simulink model "dbx_control_v0_05"  (R2015a)
settings: Solver=FixedStepDiscrete  SolverMode=SingleTasking  StartTime=0.0  StopTime=20  FixedStep=T_ctrl  RelTol=1e-3
undefined symbols (not defined in the file): A_l_max_x, A_M, A_z_max, CG, epsilon, Flaps_ang_deg, g, Hover_eta_23, Hover_throtle_1, Hover_throtle_23, I_BAC, L_M, m, psi_f_i, psi_K_b, psi_tau, Roll_pich_sens, Servo_calib, T_ctrl, Throtle_sens, v_i0, Yaw_sens
libraries: DBX_model x29, DBX_Control_lib x15, simulink x9, DBX_Control x3
(part 2 of 2)

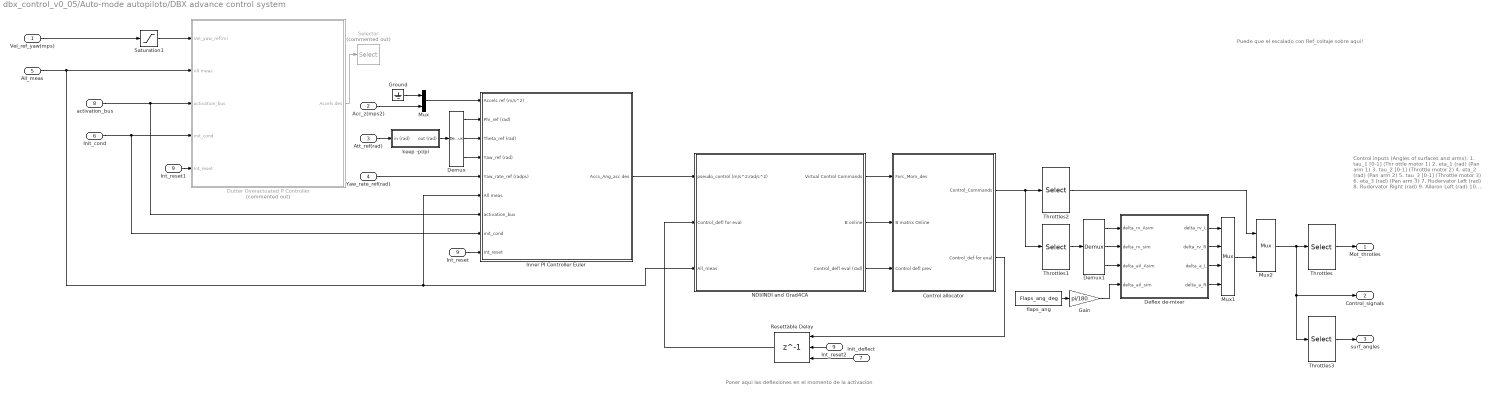
== system dbx_control_v0_05/Auto-mode autopiloto/DBX advance control system ==
  note: Puede que el escalado con Ref_coltaje sobre aqui!
  note: Poner aqui las deflexiones en el momento de la activacion
  note: Control inputs (Angles  of surfaces and arms):
      |
      | 1. tau_1 [0-1] (Thr ottle motor 1)
      | 2. eta_1 (rad)  (Pan arm 1)
      |
      | 3. tau_2 [0-1] (Throttle motor 2)
      | 4. eta_2 (rad)  (Pan arm 2)
      |
      | 5. tau_3 [0-1] (Throttle motor 3)
      | 6. eta_3 (rad)  (Pan arm  3)
      |
      | 7. Rudervator Left (rad)
      | 8. Rudervator Right (rad)
      | 9. Aileron Left (rad)
      | 10. Aielron Right (rad)
  Vel_ref_yaw(mps) : Inport
  Acc_z(mps2) : Inport  Port=2
  Att_ref(rad) : Inport  Port=3
  Yaw_rate_ref(rad) : Inport  Port=4
  All_meas : Inport  Port=5
  Init_cond : Inport  Port=6
  Init_deflect : Inport  Port=7  PortDimensions=[9,1]
  activation_bus : Inport  Port=8
  Int_reset : Inport  Port=9
  Control allocator : Subsystem  RTWFcnName=abc  RTWFileName=asas  VariantControl=Control Allocator: NO RECONFIG
      settings: MinAlgLoopOccurrences=on  RTWFcnNameOpts=User specified  RTWFileNameOpts=User specified
  Deflex de-mixer : Subsystem  TreatAsAtomicUnit=on
  Demux : Demux  Outputs=3
  Demux1 : Demux  Outputs=3
  Gain : Gain  Gain=pi/180
  Ground : Ground
  Inner PI Controller Euler : Subsystem  VariantControl=PI_quat
  Int_reset1 : InportShadow  Port=9
  Int_reset2 : InportShadow  Port=9
  Mux : Mux  Inputs=[2,1]
  Mux1 : Mux
  Mux2 : Mux  Inputs=[6,4]
  NDI/INDI and Grad4CA : Subsystem  Variant=on  VariantControl=NDI: NO RECONFIG  OverrideUsingVariant=NDI_incremental_grad
  Outter Overactuated P Controller : Subsystem  Commented=on  VariantControl=Overactuated P Controller
  Resettable Delay : Delay  DelayLength=1  InitialConditionSource=Input port  ExternalReset=Either  InputProcessing=Inherited  SampleTime=T_ctrl
      settings: InputPortMap=u0,r5,p4
  Saturation1 : Saturate  UpperLimit=[10,10,v_i0]'  LowerLimit=-[10,10,2*v_i0]'
  Selector : Selector  Commented=on  InputPortWidth=3  Indices=1:2
  Throttles : Selector  InputPortWidth=10  Indices=[1,3,5]
  Throttles1 : Selector  InputPortWidth=9  Indices=[7:9]
  Throttles2 : Selector  InputPortWidth=9  Indices=[1:6]
  Throttles3 : Selector  InputPortWidth=10  Indices=[2,4,6,7,8,9,10]
  flaps_ang : Constant  Value=Flaps_ang_deg  OutDataTypeStr=single
  keep -pi/pi : Subsystem
  Mot_throtles : Outport
  Control_signals : Outport  Port=2
  surf_angles : Outport  Port=3
  wires:
  All_meas/1 -> Inner PI Controller Euler/6(All meas), NDI/INDI and Grad4CA/3(All_meas), Outter Overactuated P Controller/2(All meas)
  NDI/INDI and Grad4CA/3(Control_defl eval (rad)) -> Control allocator/3(Control defl prev)
  keep -pi/pi/1(out (rad)) -> Demux/1
  Demux/3 -> Inner PI Controller Euler/4(Yaw_ref (rad))
  Demux/2 -> Inner PI Controller Euler/3(Theta_ref (rad))
  Demux/1 -> Inner PI Controller Euler/2(Phi_ref (rad))
  Att_ref(rad)/1 -> keep -pi/pi/1(in (rad))
  Throttles/1 -> Mot_throtles/1
  Control allocator/1(Control_Commands) -> Throttles1/1, Throttles2/1
  Resettable Delay/1 -> NDI/INDI and Grad4CA/2(Control_defl for eval)
  Vel_ref_yaw(mps)/1 -> Saturation1/1
  Saturation1/1 -> Outter Overactuated P Controller/1(Vel_yaw_ref(m))
  Init_cond/1 -> Inner PI Controller Euler/8(init_cond), Outter Overactuated P Controller/4(init_cond)
  activation_bus/1 -> Inner PI Controller Euler/7(activation_bus), Outter Overactuated P Controller/3(activation_bus)
  Control allocator/2(Control_def for eval) -> Resettable Delay/1
  NDI/INDI and Grad4CA/2(B online) -> Control allocator/2(B matrix Online)
  Inner PI Controller Euler/1(Accs_Ang_acc des) -> NDI/INDI and Grad4CA/1(pseudo_control (m/s^2;rad/s^2))
  Demux1/2 -> Deflex de-mixer/2(delta_rv_sim)
  Demux1/3 -> Deflex de-mixer/3(delta_ail_Asim)
  Demux1/1 -> Deflex de-mixer/1(delta_rv_Asim)
  Throttles1/1 -> Demux1/1
  Throttles2/1 -> Mux2/1
  Deflex de-mixer/1(delta_rv_L) -> Mux1/1
  Deflex de-mixer/2(delta_rv_R) -> Mux1/2
  Deflex de-mixer/3(delta_a_L) -> Mux1/3
  Deflex de-mixer/4(delta_a_R) -> Mux1/4
  Mux1/1 -> Mux2/2
  Mux2/1 -> Throttles3/1, Control_signals/1, Throttles/1
  Throttles3/1 -> surf_angles/1
  Yaw_rate_ref(rad)/1 -> Inner PI Controller Euler/5(Yaw_rate_ref (radps))
  Int_reset/1 -> Inner PI Controller Euler/9(Int_reset)
  Int_reset1/1 -> Outter Overactuated P Controller/5(Int_reset)
  Acc_z(mps2)/1 -> Mux/2
  Mux/1 -> Inner PI Controller Euler/1(Accels ref (m/s^2))
  Init_deflect/1 -> Resettable Delay/3
  Int_reset2/1 -> Resettable Delay/2
  NDI/INDI and Grad4CA/1(Virtual Control Commands) -> Control allocator/1(Forc_Mom_des)
  Outter Overactuated P Controller/1(Accels des) -> Selector/1
  Ground/1 -> Mux/1
  flaps_ang/1 -> Gain/1
  Gain/1 -> Deflex de-mixer/4(delta_ail_sim)

== system dbx_control_v0_05/Auto-mode autopiloto/Initial conditions ==
  All_meas : Inport
  Bus Creator1 : BusCreator  Inputs=6
  Bus Selector : BusSelector  OutputSignals=Meas.Eulr_meas_rad,Meas.omega_b_meas_radps
  Ground{,1..3} (4 alike) : Ground
  Init_cond : Outport
  wires:
  Ground2/1 -> Bus Creator1/3  "vel_yaw_xy_init"
  Bus Selector/2 -> Bus Creator1/6  "<omega_b_meas_radps>"
  Ground3/1 -> Bus Creator1/4  "vel_yaw_z_init"
  Bus Selector/1 -> Bus Creator1/5  "<Eulr_meas_rad>"
  Ground/1 -> Bus Creator1/1  "pos_xy_init"
  Ground1/1 -> Bus Creator1/2  "alt_init"
  All_meas/1 -> Bus Selector/1
  Bus Creator1/1 -> Init_cond/1

== system dbx_control_v0_05/Auto-mode autopiloto/Sensibilidades Radio ==
  Radio_in : Inport
  Demux : Demux
  Demux1 : Demux  Outputs=2
  Divide : Product  Inputs=**
  Divide1 : Product  Inputs=**
  Mux : Mux  Inputs=2
  Product : Product
  Saturation : Saturate  UpperLimit=9  LowerLimit=-5
  Throtle_sens : Constant  Value=Throtle_sens  OutDataTypeStr=single
  Unary Minus : UnaryMinus
  Yaw_sens : Constant  Value=Yaw_sens  OutDataTypeStr=single
  deg2rad : Gain  Gain=pi/180
  deg2rad1 : Gain  Gain=pi/180
  deg2rad2 : Gain  Gain=[1,-1]
  roll_pich_sens : Constant  Value=Roll_pich_sens  OutDataTypeStr=single
  Acc_z_mps2 : Outport
  Roll(rad) : Outport  Port=2
  Pitch(rad) : Outport  Port=3
  Yaw(radps) : Outport  Port=4
  wires:
  Demux/1 -> Product/1  "Throtle"
  Demux/2 -> Divide/1  "Yaw"
  Demux/3 -> Mux/2  "Pitch"
  Demux/4 -> Mux/1  "Roll"
  Radio_in/1 -> Demux/1
  Divide/1 -> Yaw(radps)/1
  Mux/1 -> Divide1/1
  Divide1/1 -> Demux1/1
  Demux1/1 -> Roll(rad)/1
  Demux1/2 -> Pitch(rad)/1
  Product/1 -> Saturation/1
  Saturation/1 -> Acc_z_mps2/1
  Yaw_sens/1 -> deg2rad/1
  deg2rad/1 -> Divide/2
  roll_pich_sens/1 -> deg2rad1/1
  deg2rad1/1 -> deg2rad2/1
  deg2rad2/1 -> Divide1/2
  Throtle_sens/1 -> Unary Minus/1
  Unary Minus/1 -> Product/2

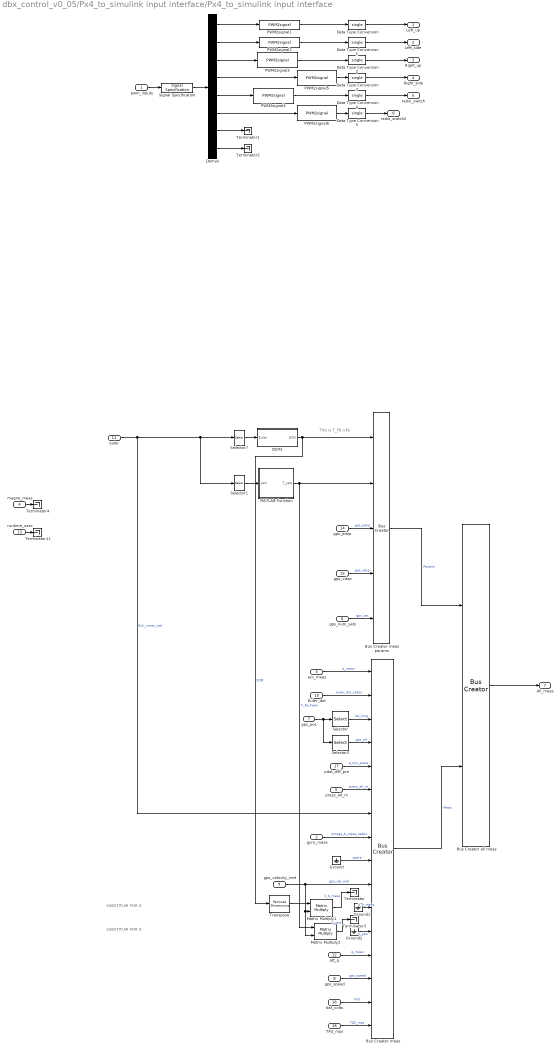
== system dbx_control_v0_05/Px4_to_simulink input interface/Px4_to_simulink input interface ==
  note: SUBSTITUIR POR 0
  note: This is T_Fb->Fe
  note: SUBSTITUIR POR 0
  pwm_inputs : Inport  PortDimensions=8  SampleTime=T_ctrl
  gyro_meas : Inport  Port=2  PortDimensions=3  SampleTime=T_ctrl
  acc_meas : Inport  Port=3  PortDimensions=3  SampleTime=T_ctrl
  magne_meas : Inport  Port=4  PortDimensions=3  SampleTime=T_ctrl
  press_alt_m : Inport  Port=5  PortDimensions=1  SampleTime=T_ctrl
  gps_num_sats : Inport  Port=6  PortDimensions=1  SampleTime=T_ctrl
  gps_pos : Inport  Port=7  PortDimensions=3  SampleTime=T_ctrl
  gps_speed : Inport  Port=8  PortDimensions=1  SampleTime=T_ctrl
  gps_velocity_ned : Inport  Port=9  PortDimensions=3  SampleTime=T_ctrl
  Euler_dot : Inport  Port=10  PortDimensions=3  SampleTime=T_ctrl
  euler : Inport  Port=11  PortDimensions=3  SampleTime=T_ctrl
  att_q : Inport  Port=12  PortDimensions=4  SampleTime=T_ctrl
  runtime_usec : Inport  Port=13  PortDimensions=1  SampleTime=T_ctrl
  gps_pdop : Inport  Port=14  PortDimensions=1  SampleTime=T_ctrl
  gps_vdop : Inport  Port=15  PortDimensions=1  SampleTime=T_ctrl
  bat_volts : Inport  Port=16  PortDimensions=1  SampleTime=T_ctrl
  pitot_diff_pre : Inport  Port=17  SampleTime=T_ctrl
  TAS_mps : Inport  Port=18  SampleTime=T_ctrl
  Bus Creator all meas : BusCreator  Inputs=2
  Bus Creator meas : BusCreator  Inputs=16
  Bus Creator meas params : BusCreator  Inputs=5
  DCM1 : Subsystem  TreatAsAtomicUnit=on
  Data Type Conversion{,1..5} (6 alike) : DataTypeConversion  OutDataTypeStr=single
  Demux : Demux  Outputs=8
  Ground : Ground
  Ground1 : Ground
  Ground2 : Ground
  MATLAB Function : MATLAB Function  TreatAsAtomicUnit=on
  Matrix Multiply1 : Product  Multiplication=Matrix(*)
  Matrix Multiply2 : Product  Multiplication=Matrix(*)
  PWM2signal{1..6} (6 alike) : DBX_model/PWM2signal  c=2000  a=1000  d=1  b=-1
  Selector : Selector  InputPortWidth=3  Indices=[1,2]
  Selector1 : Selector  InputPortWidth=3  Indices=3
  Selector2 : Selector  InputPortWidth=3  Indices=3
  Selector7 : Selector  InputPortWidth=3  Indices=[3 2 1]
  Signal Specification : SignalSpecification  Dimensions=8
  Terminator{,1..4,11} (6 alike) : Terminator
  Transpose : PermuteDimensions
  Left_up : Outport
  Left_side : Outport  Port=2
  Right_up : Outport  Port=3
  Right_side : Outport  Port=4
  radio_switch : Outport  Port=5
  radio_siwtch2 : Outport  Port=6
  All_meas : Outport  Port=7
  wires:
  PWM2signal1/1 -> Data Type Conversion/1
  PWM2signal2/1 -> Data Type Conversion1/1
  PWM2signal3/1 -> Data Type Conversion2/1
  PWM2signal5/1 -> Data Type Conversion3/1
  Bus Creator all meas/1 -> All_meas/1
  PWM2signal4/1 -> Data Type Conversion4/1
  att_q/1 -> Bus Creator meas/13  "q_meas"
  euler/1 -> Bus Creator meas/7, Selector1/1, Selector7/1  "Eulr_meas_rad"
  Euler_dot/1 -> Bus Creator meas/2  "euler_dot_radps"
  bat_volts/1 -> Bus Creator meas/15  "Volt"
  Bus Creator meas/1 -> Bus Creator all meas/2  "Meas"
  Bus Creator meas params/1 -> Bus Creator all meas/1  "Params"
  DCM1/1(DCM) -> Transpose/1, Bus Creator meas params/1  "DCM"
  acc_meas/1 -> Bus Creator meas/1  "a_meas"
  gps_pdop/1 -> Bus Creator meas params/3  "gps_pdop"
  gps_num_sats/1 -> Bus Creator meas params/5  "gps_sat"
  gps_vdop/1 -> Bus Creator meas params/4  "gps_vdop"
  Selector7/1 -> DCM1/1(Euler)
  Selector1/1 -> MATLAB Function/1(yaw)
  MATLAB Function/1(T_yaw) -> Matrix Multiply2/1, Bus Creator meas params/2  "T_Fe_Fyaw"
  Demux/1 -> PWM2signal1/1
  Demux/2 -> PWM2signal2/1
  Demux/3 -> PWM2signal3/1
  Demux/4 -> PWM2signal5/1
  Demux/5 -> PWM2signal4/1
  pwm_inputs/1 -> Signal Specification/1
  Demux/6 -> PWM2signal6/1
  Demux/7 -> Terminator1/1
  Demux/8 -> Terminator2/1
  gyro_meas/1 -> Bus Creator meas/8  "omega_b_meas_radps"
  magne_meas/1 -> Terminator4/1
  press_alt_m/1 -> Bus Creator meas/6  "press_alt_m"
  gps_pos/1 -> Selector2/1, Selector/1
  gps_speed/1 -> Bus Creator meas/14  "gps_speed"
  gps_velocity_ned/1 -> Bus Creator meas/10, Matrix Multiply1/2, Matrix Multiply2/2  "gps_vel_ned"
  runtime_usec/1 -> Terminator11/1
  Signal Specification/1 -> Demux/1
  PWM2signal6/1 -> Data Type Conversion5/1
  pitot_diff_pre/1 -> Bus Creator meas/5  "q_dyn_press"
  Selector/1 -> Bus Creator meas/3  "lat_long"
  Selector2/1 -> Bus Creator meas/4  "gps_alt"
  TAS_mps/1 -> Bus Creator meas/16  "TAS_mps"
  Transpose/1 -> Matrix Multiply1/1
  Ground1/1 -> Bus Creator meas/11  "V_b_meas"
  Ground2/1 -> Bus Creator meas/12  "V_yaw"
  Ground/1 -> Bus Creator meas/9  "spare"
  Matrix Multiply1/1 -> Terminator/1  "V_b_meas"
  Matrix Multiply2/1 -> Terminator3/1  "V_yaw"
  Data Type Conversion/1 -> Left_up/1
  Data Type Conversion1/1 -> Left_side/1
  Data Type Conversion2/1 -> Right_up/1
  Data Type Conversion3/1 -> Right_side/1
  Data Type Conversion4/1 -> radio_switch/1
  Data Type Conversion5/1 -> radio_siwtch2/1

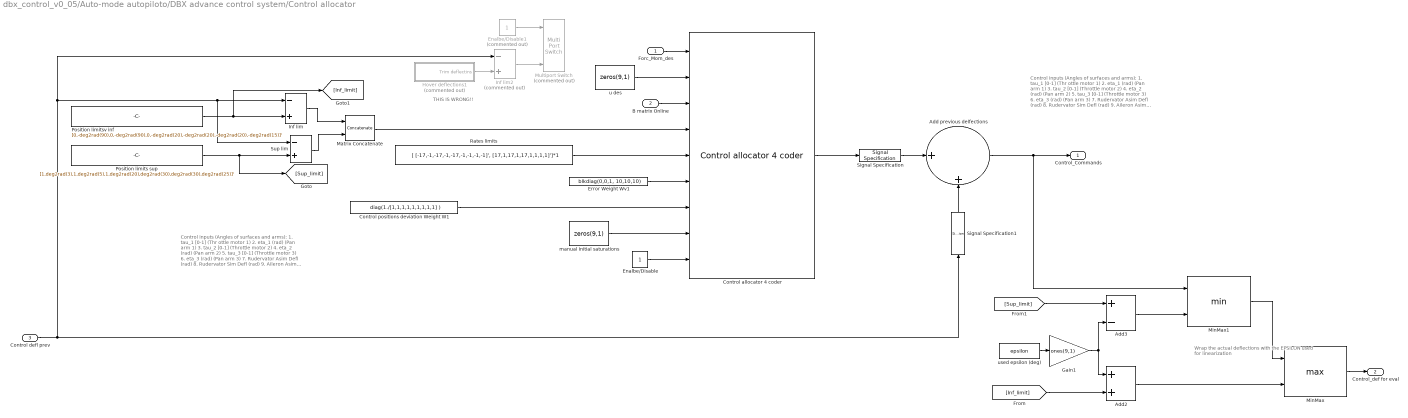
== system dbx_control_v0_05/Auto-mode autopiloto/DBX advance control system/Control allocator ==
  note: THIS IS WRONG!!
  note: Wrap the actual deflections with the EPSILON
      |  used for linearization
  note: Control inputs (Angles  of surfaces and arms):
      |
      | 1. tau_1 [0-1] (Thr ottle motor 1)
      | 2. eta_1 (rad)  (Pan arm 1)
      |
      | 3. tau_2 [0-1] (Throttle motor 2)
      | 4. eta_2 (rad)  (Pan arm 2)
      |
      | 5. tau_3 [0-1] (Throttle motor 3)
      | 6. eta_3 (rad)  (Pan arm  3)
      |
      | 7. Rudervator Asim Defl (rad)
      | 8. Rudervator Sim Defl (rad)
      | 9. Aileron Asim Defl (rad)
  note: Control inputs (Angles  of surfaces and arms):
      |
      | 1. tau_1 [0-1] (Thr ottle motor 1)
      | 2. eta_1 (rad)  (Pan arm 1)
      |
      | 3. tau_2 [0-1] (Throttle motor 2)
      | 4. eta_2 (rad)  (Pan arm 2)
      |
      | 5. tau_3 [0-1] (Throttle motor 3)
      | 6. eta_3 (rad)  (Pan arm  3)
      |
      | 7. Rudervator Asim Defl (rad)
      | 8. Rudervator Sim Defl (rad)
      | 9. Aileron Asim Defl (rad)
  Forc_Mom_des : Inport
  B matrix Online : Inport  Port=2
  Control defl prev : Inport  Port=3
  Add previous delfections : Sum  Inputs=|++
  Add2 : Sum
  Add3 : Sum  Inputs=+-
  Control allocator 4 coder : DBX_Control_lib/Control allocator 4 coder  gamma=1  imax=20  T=T_ctrl
  Control positions deviation Weight W1 : Constant  Value=diag(1./[1,1,1,1,1,1,1,1,1] )  OutDataTypeStr=single
  Enalbe/Disable : Constant  OutDataTypeStr=single
  Enalbe/Disable1 : Constant  Commented=on
  Error Weight Wv1 : Constant  Value=blkdiag(0,0,1, 10,10,10)  OutDataTypeStr=single
  Gain1 : Gain  Gain=ones(9,1)
  Hover deflections1 : Subsystem  Commented=on  TreatAsAtomicUnit=on
  Inf lim : Sum  Inputs=-+
  Inf lim2 : Sum  Commented=on  Inputs=-+
  Matrix Concatenate : Concatenate  Mode=Multidimensional array  ConcatenateDimension=2
  MinMax : MinMax  Function=max  Inputs=2
  MinMax1 : MinMax  Inputs=2
  Multiport Switch : MultiPortSwitch  Commented=on  Inputs=2
  Position limits sup : Constant  Value=[1,deg2rad(3),1,deg2rad(5),1,deg2rad(20),deg2rad(30),deg2rad(30),deg2rad(25)]'  OutDataTypeStr=single
  Position limitsv inf : Constant  Value=[0,-deg2rad(90),0,-deg2rad(90),0,-deg2rad(20),-deg2rad(20),-deg2rad(20),-deg2rad(15)]'  OutDataTypeStr=single
  Rates limits : Constant  Value=[ [-17,-1,-17,-1,-17,-1,-1,-1,-1]', [17,1,17,1,17,1,1,1,1]']*1  OutDataTypeStr=single
  Signal Specification : SignalSpecification  OutDataTypeStr=single  Dimensions=[9,1]
  Signal Specification1 : SignalSpecification  OutDataTypeStr=single  Dimensions=[9,1]
  Sup lim : Sum  Inputs=-+
  manual Initial saturations : Constant  Value=zeros(9,1)  OutDataTypeStr=single
  u des : Constant  Value=zeros(9,1)  OutDataTypeStr=single
  used epsilon (deg) : Constant  Value=epsilon  OutDataTypeStr=single
  Control_Commands : Outport
  Control_def for eval : Outport  Port=2
  wires:
  MinMax1/1 -> MinMax/1
  Add3/1 -> MinMax1/2
  used epsilon (deg)/1 -> Gain1/1
  Gain1/1 -> Add3/2, Add2/1
  Add2/1 -> MinMax/2
  Control positions deviation Weight W1/1 -> Control allocator 4 coder/7
  Control allocator 4 coder/1 -> Signal Specification/1
  Enalbe/Disable/1 -> Control allocator 4 coder/9
  manual Initial saturations/1 -> Control allocator 4 coder/8
  Sup lim/1 -> Matrix Concatenate/2
  Inf lim/1 -> Matrix Concatenate/1
  Position limitsv inf/1 -> [Inf_limit], Inf lim/2
  Position limits sup/1 -> [Sup_limit], Sup lim/2
  Rates limits/1 -> Control allocator 4 coder/5
  Add previous delfections/1 -> Control_Commands/1, MinMax1/1
  B matrix Online/1 -> Control allocator 4 coder/3
  Signal Specification/1 -> Add previous delfections/1
  Signal Specification1/1 -> Add previous delfections/2
  Forc_Mom_des/1 -> Control allocator 4 coder/1
  Matrix Concatenate/1 -> Control allocator 4 coder/4
  Control defl prev/1 -> Inf lim2/1, Inf lim/1, Sup lim/1, Signal Specification1/1
  Inf lim2/1 -> Multiport Switch/3
  Hover deflections1/1(Trim deflectins) -> Inf lim2/2
  MinMax/1 -> Control_def for eval/1
  Error Weight Wv1/1 -> Control allocator 4 coder/6
  [Inf_limit] -> Add2/2
  [Sup_limit] -> Add3/1
  Enalbe/Disable1/1 -> Multiport Switch/1
  u des/1 -> Control allocator 4 coder/2

== system dbx_control_v0_05/Auto-mode autopiloto/DBX advance control system/Deflex de-mixer ==
  note: Control outputs:
      |
      | 7. Rudervator Left (rad)
      | 8. Rudervator Right (rad)
      | 9. Aileron Left (rad)
      | 10. Aielron Right (rad)
  delta_rv_Asim : Inport
  delta_rv_sim : Inport  Port=2
  delta_ail_Asim : Inport  Port=3
  delta_ail_sim : Inport  Port=4
  Add : Sum  Inputs=|++
  Add1 : Sum  Inputs=|-+
  Add2 : Sum  Inputs=|++
  Add3 : Sum  Inputs=|-+
  delta_rv_L : Outport
  delta_rv_R : Outport  Port=2
  delta_a_L : Outport  Port=3
  delta_a_R : Outport  Port=4
  wires:
  delta_rv_Asim/1 -> Add1/1, Add/1
  Add/1 -> delta_rv_L/1
  delta_rv_sim/1 -> Add1/2, Add/2
  Add1/1 -> delta_rv_R/1
  delta_ail_Asim/1 -> Add3/1, Add2/1
  Add2/1 -> delta_a_L/1
  delta_ail_sim/1 -> Add2/2, Add3/2
  Add3/1 -> delta_a_R/1

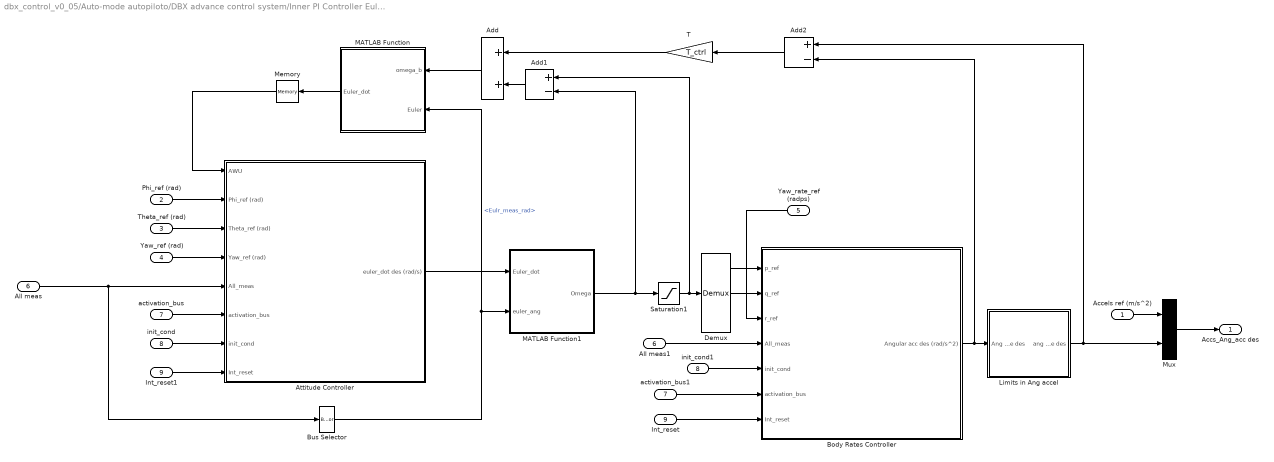
== system dbx_control_v0_05/Auto-mode autopiloto/DBX advance control system/Inner PI Controller Euler ==
  Accels ref (m/s^2) : Inport
  Phi_ref (rad) : Inport  Port=2
  Theta_ref (rad) : Inport  Port=3
  Yaw_ref (rad) : Inport  Port=4
  Yaw_rate_ref (radps) : Inport  Port=5
  All meas : Inport  Port=6
  activation_bus : Inport  Port=7
  init_cond : Inport  Port=8
  Int_reset : Inport  Port=9
  Add : Sum
  Add1 : Sum  Inputs=+-
  Add2 : Sum  Inputs=+-
  All meas1 : InportShadow  Port=6
  Attitude Controller : Subsystem
  Body Rates Controller : Subsystem
  Bus Selector : BusSelector  OutputSignals=Meas.Eulr_meas_rad
  Demux : Demux  Outputs=3
  Int_reset1 : InportShadow  Port=9
  Limits in Ang accel : Subsystem
  MATLAB Function : MATLAB Function
  MATLAB Function1 : MATLAB Function
  Memory : Memory
  Mux : Mux  Inputs=2
  Saturation1 : Saturate  UpperLimit=deg2rad(400)*[1,1,1]'  LowerLimit=-deg2rad(400)*[1,1,1]'
  T : Gain  Gain=T_ctrl
  activation_bus1 : InportShadow  Port=7
  init_cond1 : InportShadow  Port=8
  Accs_Ang_acc des : Outport
  wires:
  Accels ref (m/s^2)/1 -> Mux/1
  Mux/1 -> Accs_Ang_acc des/1
  All meas/1 -> Bus Selector/1, Attitude Controller/5(All_meas)
  Bus Selector/1 -> MATLAB Function/2(Euler), MATLAB Function1/2(euler_ang)  "<Eulr_meas_rad>"
  Demux/1 -> Body Rates Controller/1(p_ref)
  Demux/2 -> Body Rates Controller/2(q_ref)
  Phi_ref (rad)/1 -> Attitude Controller/2(Phi_ref (rad))
  Yaw_ref (rad)/1 -> Attitude Controller/4(Yaw_ref (rad))
  Limits in Ang accel/1(ang Ace des) -> Add2/1, Mux/2
  MATLAB Function1/1(Omega) -> Add1/2, Saturation1/1
  Body Rates Controller/1(Angular acc des (rad/s^2)) -> Add2/2, Limits in Ang accel/1(Ang Ace des)
  Add/1 -> MATLAB Function/1(omega_b)
  Add2/1 -> T/1
  Add1/1 -> Add/2
  T/1 -> Add/1
  MATLAB Function/1(Euler_dot) -> Memory/1
  init_cond/1 -> Attitude Controller/7(init_cond)
  activation_bus/1 -> Attitude Controller/6(activation_bus)
  All meas1/1 -> Body Rates Controller/4(All_meas)
  Saturation1/1 -> Add1/1, Demux/1
  Memory/1 -> Attitude Controller/1(AWU)
  Theta_ref (rad)/1 -> Attitude Controller/3(Theta_ref (rad))
  Attitude Controller/1(euler_dot des (rad/s)) -> MATLAB Function1/1(Euler_dot)
  Int_reset/1 -> Body Rates Controller/7(Int_reset)
  Int_reset1/1 -> Attitude Controller/8(Int_reset)
  activation_bus1/1 -> Body Rates Controller/6(activation_bus)
  init_cond1/1 -> Body Rates Controller/5(init_cond)
  Yaw_rate_ref (radps)/1 -> Body Rates Controller/3(r_ref)

== system dbx_control_v0_05/Auto-mode autopiloto/DBX advance control system/NDI//INDI and Grad4CA ==
  pseudo_control (m/s^2;rad/s^2) : Inport
  Control_defl for eval : Inport  Port=2
  All_meas : Inport  Port=3
  INDI and NDI : Subsystem  RTWFcnName=abc  RTWFileName=asas  VariantControl=NDI_INDI
      settings: RTWFcnNameOpts=User specified  RTWFileNameOpts=User specified
  NDI : Subsystem  RTWFcnName=abc  RTWFileName=asas  VariantControl=NDI
      settings: RTWFcnNameOpts=User specified  RTWFileNameOpts=User specified
  NDI incremental gradient : Subsystem  RTWFcnName=abc  RTWFileName=asas  VariantControl=NDI_incremental_grad
      settings: RTWFcnNameOpts=User specified  RTWFileNameOpts=User specified
  Virtual Control Commands : Outport
  B online : Outport  Port=2
  Control_defl eval (rad) : Outport  Port=3

== system dbx_control_v0_05/Auto-mode autopiloto/DBX advance control system/Outter Overactuated P Controller ==
  Vel_yaw_ref(m) : Inport
  All meas : Inport  Port=2
  activation_bus : Inport  Port=3
  init_cond : Inport  Port=4
  Int_reset : Inport  Port=5
  Bus Selector1 : BusSelector  OutputSignals=Params.T_Fe_Fyaw,Meas.V_yaw,Params.DCM
  Demux2 : Demux  Outputs=3
  Matrix Multiply1 : Product  Multiplication=Matrix(*)
  Matrix Multiply3 : Product  Multiplication=Matrix(*)
  Permute Dimensions : PermuteDimensions
  Permute Dimensions1 : PermuteDimensions
  Saturation : Saturate  UpperLimit=[A_l_max_x,10,g]  LowerLimit=-[A_l_max_x,10,A_z_max-g]
  Saturation1 : Saturate  UpperLimit=[10,10,v_i0]'  LowerLimit=-[10,10,2*v_i0]'
  Terminator : Terminator
  Velocity Controller : Subsystem
  Accels des : Outport
  wires:
  Demux2/3 -> Velocity Controller/2(Vyaw_z_ref)
  Demux2/1 -> Velocity Controller/1(Vyaw_x_ref)
  All meas/1 -> Bus Selector1/1
  Bus Selector1/3 -> Permute Dimensions/1  "<DCM>"
  Matrix Multiply1/1 -> Accels des/1
  Permute Dimensions/1 -> Matrix Multiply1/1
  Saturation1/1 -> Demux2/1
  Saturation/1 -> Matrix Multiply3/2
  Bus Selector1/1 -> Permute Dimensions1/1  "<T_Fe_Fyaw>"
  Vel_yaw_ref(m)/1 -> Saturation1/1
  Matrix Multiply3/1 -> Matrix Multiply1/2  "in F_e"
  Permute Dimensions1/1 -> Matrix Multiply3/1
  Velocity Controller/1(Acc_yaw des (m/s)) -> Saturation/1
  activation_bus/1 -> Velocity Controller/4(activation_bus)
  Bus Selector1/2 -> Velocity Controller/3(V_yaw_meas)  "<V_yaw>"
  init_cond/1 -> Velocity Controller/5(Init_cond)
  Demux2/2 -> Terminator/1
  Int_reset/1 -> Velocity Controller/6(Int_reset)

== system dbx_control_v0_05/Auto-mode autopiloto/DBX advance control system/keep -pi//pi ==
  in (rad) : Inport  OutDataTypeStr=single
  Constant : Constant  Value=180  OutDataTypeStr=single
  Constant2 : Constant  Value=360  OutDataTypeStr=single
  Gain : Gain  Gain=360
  Math Function2 : Math  Operator=rem  SaturateOnIntegerOverflow=on
  Product : Product  Inputs=*/  RndMeth=Zero
  Rounding Function : Rounding  Operator=fix
  Sum2 : Sum  Inputs=|-+
  deg2rad1 : Gain  Gain=pi/180  SaturateOnIntegerOverflow=on  OutDataTypeStr=Inherit: Same as input  ParamDataTypeStr=Inherit: Same as input
  rad2deg : Gain  Gain=180/pi  SaturateOnIntegerOverflow=on  OutDataTypeStr=Inherit: Same as input  ParamDataTypeStr=Inherit: Same as input
  out (rad) : Outport
  wires:
  deg2rad1/1 -> out (rad)/1
  Sum2/1 -> deg2rad1/1
  Math Function2/1 -> Sum2/2, Product/1
  Constant2/1 -> Math Function2/2
  rad2deg/1 -> Math Function2/1
  Gain/1 -> Sum2/1
  Rounding Function/1 -> Gain/1
  Product/1 -> Rounding Function/1
  Constant/1 -> Product/2
  in (rad)/1 -> rad2deg/1

== system dbx_control_v0_05/Px4_to_simulink input interface/Px4_to_simulink input interface/DCM1 ==
  Euler : Inport  PortDimensions=3
  Fcn11 : Fcn  Expr=u(5)*u(4)
  Fcn12 : Fcn  Expr=u(5)*u(1)
  Fcn13 : Fcn  Expr=-u(2)
  Fcn21 : Fcn  Expr=u(3)*u(2)*u(4) - u(6)*u(1)
  Fcn22 : Fcn  Expr=u(3)*u(2)*u(1) + u(6)*u(4)
  Fcn23 : Fcn  Expr=u(3)*u(5)
  Fcn31 : Fcn  Expr=u(6)*u(2)*u(4) + u(3)*u(1)
  Fcn32 : Fcn  Expr=u(6)*u(2)*u(1) - u(3)*u(4)
  Fcn33 : Fcn  Expr=u(6)*u(5)
  Mux : Mux  Inputs=2
  Mux1 : Mux  Inputs=9
  Reshape : Reshape  OutputDimensionality=Customize  OutputDimensions=[3,3]
  sincos : Trigonometry  Operator=sincos
  DCM : Outport  PortDimensions=[3,3]
  wires:
  Fcn33/1 -> Mux1/9
  Fcn32/1 -> Mux1/8
  Fcn23/1 -> Mux1/6
  Fcn22/1 -> Mux1/5
  Fcn31/1 -> Mux1/7
  Fcn21/1 -> Mux1/4
  Fcn13/1 -> Mux1/3
  Fcn12/1 -> Mux1/2
  Fcn11/1 -> Mux1/1
  Mux/1 -> Fcn22/1, Fcn23/1, Fcn31/1, Fcn33/1, Fcn32/1, Fcn21/1, Fcn13/1, Fcn12/1, Fcn11/1
  sincos/2 -> Mux/2
  sincos/1 -> Mux/1
  Reshape/1 -> DCM/1
  Euler/1 -> sincos/1
  Mux1/1 -> Reshape/1

== system dbx_control_v0_05/Auto-mode autopiloto/DBX advance control system/Control allocator/Hover deflections1 ==
  Contro Inputs1 : Constant  Value=Hover_throtle_1
  Contro Inputs2 : Constant  Value=Hover_throtle_23
  Contro Inputs3 : Constant  Value=Hover_eta_23
  Gain : Gain  Gain=-1
  Ground : Ground
  Mux : Mux  Inputs=9
  Trim deflectins : Outport
  wires:
  Contro Inputs1/1 -> Mux/1
  Contro Inputs2/1 -> Mux/7, Mux/4
  Ground/1 -> Mux/2, Mux/6, Mux/9, Mux/3
  Contro Inputs3/1 -> Gain/1, Mux/5
  Gain/1 -> Mux/8
  Mux/1 -> Trim deflectins/1

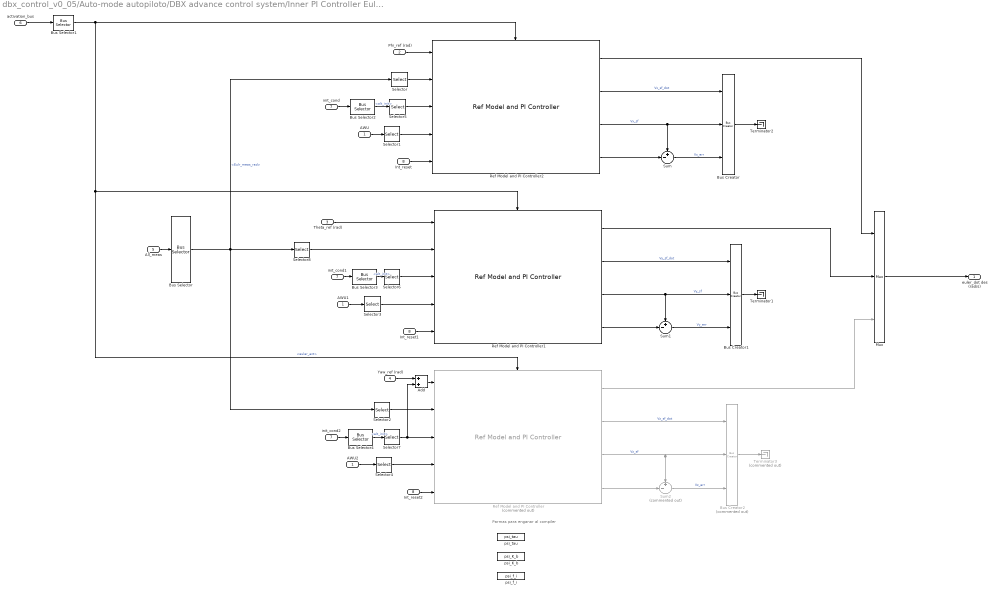
== system dbx_control_v0_05/Auto-mode autopiloto/DBX advance control system/Inner PI Controller Euler/Attitude Controller ==
  note: Parmas para enganar al compiler
  AWU : Inport
  Phi_ref (rad) : Inport  Port=2
  Theta_ref (rad) : Inport  Port=3
  Yaw_ref (rad) : Inport  Port=4
  All_meas : Inport  Port=5
  activation_bus : Inport  Port=6
  init_cond : Inport  Port=7
  Int_reset : Inport  Port=8
  AWU1 : InportShadow
  AWU2 : InportShadow
  Add : Sum
  Bus Creator : BusCreator  Inputs=3
  Bus Creator1 : BusCreator  Inputs=3
  Bus Creator2 : BusCreator  Commented=on  Inputs=3
  Bus Selector : BusSelector  OutputSignals=Meas.Eulr_meas_rad
  Bus Selector1 : BusSelector  OutputSignals=euler_act
  Bus Selector2 : BusSelector  OutputSignals=alt_init
  Bus Selector3 : BusSelector  OutputSignals=alt_init
  Bus Selector4 : BusSelector  OutputSignals=alt_init
  Int_reset1 : InportShadow  Port=8
  Int_reset2 : InportShadow  Port=8
  Mux : Mux  Inputs=3
  Ref Model and PI Controller : DBX_Control_lib/Ref Model and PI Controller  Commented=on  delta=0  tau=psi_tau  RisingSlewLimit=deg2rad(400)  FallingSlewLimit=-deg2rad(400)  K_f=0.2  K_a=1  Con_way=pro  omega_n=4  xi=0.5  Z1=-30  K_b=psi_K_b  f_i=psi_f_i  f_c=1
  Ref Model and PI Controller1 : DBX_Control_lib/Ref Model and PI Controller  delta=0  tau=theta_tau  RisingSlewLimit=deg2rad(400)  FallingSlewLimit=-deg2rad(400)  K_f=1  K_a=1  Con_way=pro  omega_n=4  xi=0.5  Z1=-30  K_b=theta_K_b  f_i=theta_f_i  f_c=1
  Ref Model and PI Controller2 : DBX_Control_lib/Ref Model and PI Controller  delta=0  tau=phi_tau  RisingSlewLimit=deg2rad(40)  FallingSlewLimit=-deg2rad(40)  K_f=1  K_a=1  Con_way=pro  omega_n=4  xi=0.6  Z1=-30  K_b=phi_K_b  f_i=phi_f_i  f_c=1
  Selector : Selector  InputPortWidth=3
  Selector1 : Selector  InputPortWidth=3
  Selector2 : Selector  InputPortWidth=3  Indices=3
  Selector3 : Selector  InputPortWidth=3  Indices=2
  Selector4 : Selector  InputPortWidth=3  Indices=3
  Selector5 : Selector  InputPortWidth=3
  Selector6 : Selector  InputPortWidth=3  Indices=2
  Selector7 : Selector  InputPortWidth=3  Indices=3
  Selector8 : Selector  InputPortWidth=3  Indices=2
  Sum : Sum  Inputs=+-|
  Sum1 : Sum  Inputs=+-|
  Sum2 : Sum  Commented=on  Inputs=+-|
  Terminator1 : Terminator
  Terminator2 : Terminator
  Terminator3 : Terminator  Commented=on
  init_cond1 : InportShadow  Port=7
  init_cond2 : InportShadow  Port=7
  psi_K_b : Constant  Value=psi_K_b  OutDataTypeStr=single
  psi_f_i : Constant  Value=psi_f_i  OutDataTypeStr=single
  psi_tau : Constant  Value=psi_tau  OutDataTypeStr=single
  euler_dot des (rad/s) : Outport
  wires:
  Ref Model and PI Controller/4 -> Sum2/2
  Sum2/1 -> Bus Creator2/3  "Vz_err"
  Ref Model and PI Controller/3 -> Bus Creator2/2, Sum2/1  "Vz_sf"
  Ref Model and PI Controller/2 -> Bus Creator2/1  "Vz_sf_dot"
  Ref Model and PI Controller1/4 -> Sum1/2
  Sum1/1 -> Bus Creator1/3  "Vy_err"
  Ref Model and PI Controller1/3 -> Sum1/1, Bus Creator1/2  "Vy_sf"
  Ref Model and PI Controller1/2 -> Bus Creator1/1  "Vy_sf_dot"
  Ref Model and PI Controller2/4 -> Sum/2
  Bus Creator2/1 -> Terminator3/1
  Bus Creator1/1 -> Terminator1/1
  Bus Creator/1 -> Terminator2/1
  Sum/1 -> Bus Creator/3  "Vx_err"
  Ref Model and PI Controller2/3 -> Sum/1, Bus Creator/2  "Vx_sf"
  Ref Model and PI Controller2/2 -> Bus Creator/1  "Vx_sf_dot"
  Yaw_ref (rad)/1 -> Add/1
  Selector/1 -> Ref Model and PI Controller2/2
  All_meas/1 -> Bus Selector/1
  Phi_ref (rad)/1 -> Ref Model and PI Controller2/1
  Mux/1 -> euler_dot des (rad/s)/1
  Ref Model and PI Controller2/1 -> Mux/1
  Ref Model and PI Controller/1 -> Mux/3
  Ref Model and PI Controller1/1 -> Mux/2
  Selector2/1 -> Ref Model and PI Controller/2
  Bus Selector/1 -> Selector2/1, Selector/1, Selector8/1  "<Eulr_meas_rad>"
  Selector8/1 -> Ref Model and PI Controller1/2
  Theta_ref (rad)/1 -> Ref Model and PI Controller1/1
  AWU/1 -> Selector1/1
  AWU1/1 -> Selector3/1
  AWU2/1 -> Selector4/1
  Selector1/1 -> Ref Model and PI Controller2/4
  Selector3/1 -> Ref Model and PI Controller1/4
  Selector4/1 -> Ref Model and PI Controller/4
  activation_bus/1 -> Bus Selector1/1
  Bus Selector1/1 -> Ref Model and PI Controller/Enable, Ref Model and PI Controller1/Enable, Ref Model and PI Controller2/Enable  "<euler_act>"
  init_cond/1 -> Bus Selector2/1
  Bus Selector2/1 -> Selector5/1  "<alt_init>"
  Selector5/1 -> Ref Model and PI Controller2/3
  Selector6/1 -> Ref Model and PI Controller1/3
  init_cond1/1 -> Bus Selector3/1
  Bus Selector3/1 -> Selector6/1  "<alt_init>"
  init_cond2/1 -> Bus Selector4/1
  Selector7/1 -> Ref Model and PI Controller/3, Add/2
  Bus Selector4/1 -> Selector7/1  "<alt_init>"
  Int_reset/1 -> Ref Model and PI Controller2/5
  Int_reset1/1 -> Ref Model and PI Controller1/5
  Int_reset2/1 -> Ref Model and PI Controller/5
  Add/1 -> Ref Model and PI Controller/1

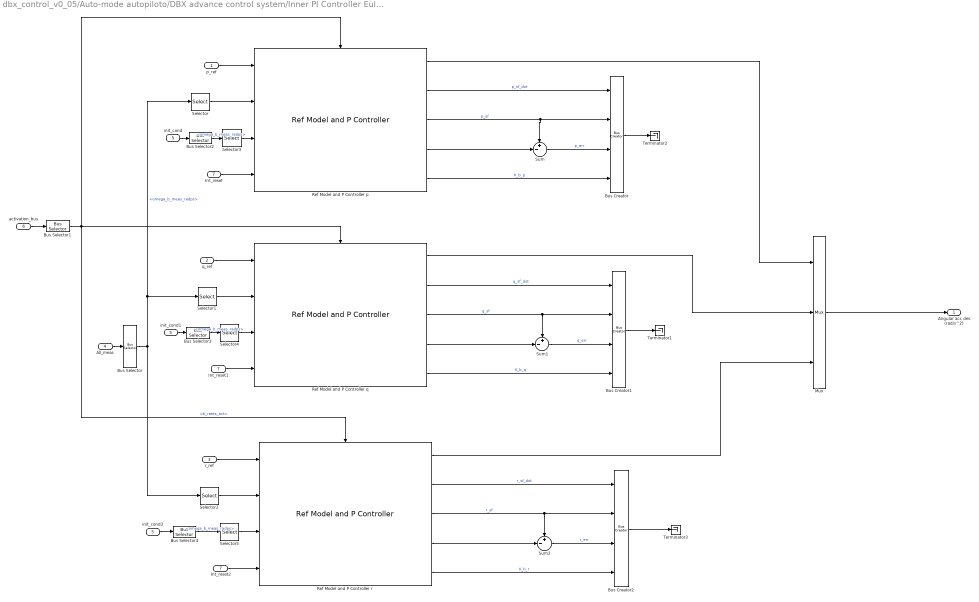
== system dbx_control_v0_05/Auto-mode autopiloto/DBX advance control system/Inner PI Controller Euler/Body Rates Controller ==
  p_ref : Inport
  q_ref : Inport  Port=2
  r_ref : Inport  Port=3
  All_meas : Inport  Port=4
  init_cond : Inport  Port=5
  activation_bus : Inport  Port=6
  Int_reset : Inport  Port=7
  Bus Creator : BusCreator
  Bus Creator1 : BusCreator
  Bus Creator2 : BusCreator
  Bus Selector : BusSelector  OutputSignals=Meas.omega_b_meas_radps
  Bus Selector1 : BusSelector  OutputSignals=b_rates_act
  Bus Selector2 : BusSelector  OutputSignals=omega_b_meas_radps
  Bus Selector3 : BusSelector  OutputSignals=omega_b_meas_radps
  Bus Selector4 : BusSelector  OutputSignals=omega_b_meas_radps
  Int_reset1 : InportShadow  Port=7
  Int_reset2 : InportShadow  Port=7
  Mux : Mux  Inputs=3
  Ref Model and P Controller p : DBX_Control_lib/Ref Model and P Controller  tau=p_tau  RisingSlewLimit=40  FallingSlewLimit=-40  K_f=1  K_b=p_K_b
  Ref Model and P Controller q : DBX_Control_lib/Ref Model and P Controller  tau=q_tau  RisingSlewLimit=40  FallingSlewLimit=-40  K_f=1  K_b=q_K_b
  Ref Model and P Controller r : DBX_Control_lib/Ref Model and P Controller  tau=r_tau  RisingSlewLimit=40  FallingSlewLimit=-40  K_f=0.6  K_b=r_K_b
  Selector : Selector  InputPortWidth=3
  Selector1 : Selector  InputPortWidth=3  Indices=2
  Selector2 : Selector  InputPortWidth=3  Indices=3
  Selector3 : Selector  InputPortWidth=3
  Selector4 : Selector  InputPortWidth=3  Indices=2
  Selector5 : Selector  InputPortWidth=3  Indices=[3]
  Sum : Sum  Inputs=+-|
  Sum1 : Sum  Inputs=+-|
  Sum2 : Sum  Inputs=+-|
  Terminator1 : Terminator
  Terminator2 : Terminator
  Terminator3 : Terminator
  init_cond1 : InportShadow  Port=5
  init_cond2 : InportShadow  Port=5
  Angular acc des (rad/s^2) : Outport
  wires:
  Ref Model and P Controller r/5 -> Bus Creator2/4  "K_b_r"
  Ref Model and P Controller r/4 -> Sum2/2
  Sum2/1 -> Bus Creator2/3  "r_err"
  Ref Model and P Controller r/3 -> Bus Creator2/2, Sum2/1  "r_sf"
  Ref Model and P Controller r/2 -> Bus Creator2/1  "r_sf_dot"
  Ref Model and P Controller q/5 -> Bus Creator1/4  "K_b_q"
  Ref Model and P Controller q/4 -> Sum1/2
  Sum1/1 -> Bus Creator1/3  "q_err"
  Ref Model and P Controller q/3 -> Bus Creator1/2, Sum1/1  "q_sf"
  Ref Model and P Controller q/2 -> Bus Creator1/1  "q_sf_dot"
  Ref Model and P Controller p/5 -> Bus Creator/4  "K_b_p"
  Ref Model and P Controller p/4 -> Sum/2
  Selector2/1 -> Ref Model and P Controller r/2
  Bus Creator2/1 -> Terminator3/1
  Bus Creator1/1 -> Terminator1/1
  Bus Creator/1 -> Terminator2/1
  Sum/1 -> Bus Creator/3  "p_err"
  Ref Model and P Controller p/3 -> Bus Creator/2, Sum/1  "p_sf"
  Ref Model and P Controller p/2 -> Bus Creator/1  "p_sf_dot"
  r_ref/1 -> Ref Model and P Controller r/1
  Selector1/1 -> Ref Model and P Controller q/2
  q_ref/1 -> Ref Model and P Controller q/1
  Mux/1 -> Angular acc des (rad/s^2)/1
  p_ref/1 -> Ref Model and P Controller p/1
  Bus Selector/1 -> Selector2/1, Selector/1, Selector1/1  "<omega_b_meas_radps>"
  All_meas/1 -> Bus Selector/1
  Ref Model and P Controller r/1 -> Mux/3
  Ref Model and P Controller q/1 -> Mux/2
  Ref Model and P Controller p/1 -> Mux/1
  Selector/1 -> Ref Model and P Controller p/2
  activation_bus/1 -> Bus Selector1/1
  Bus Selector1/1 -> Ref Model and P Controller p/Enable, Ref Model and P Controller r/Enable, Ref Model and P Controller q/Enable  "<b_rates_act>"
  init_cond/1 -> Bus Selector2/1
  Bus Selector2/1 -> Selector3/1  "<omega_b_meas_radps>"
  Selector3/1 -> Ref Model and P Controller p/3
  init_cond1/1 -> Bus Selector3/1
  Bus Selector3/1 -> Selector4/1  "<omega_b_meas_radps>"
  Selector4/1 -> Ref Model and P Controller q/3
  init_cond2/1 -> Bus Selector4/1
  Bus Selector4/1 -> Selector5/1  "<omega_b_meas_radps>"
  Selector5/1 -> Ref Model and P Controller r/3
  Int_reset/1 -> Ref Model and P Controller p/4
  Int_reset1/1 -> Ref Model and P Controller q/4
  Int_reset2/1 -> Ref Model and P Controller r/4

== system dbx_control_v0_05/Auto-mode autopiloto/DBX advance control system/Inner PI Controller Euler/Limits in Ang accel ==
  note: Here it is assumed that at all time every prop is generating m*g/3 newtons of force . It is conservative?
  Ang Ace des : Inport
  Data Type Conversion1 : DataTypeConversion  OutDataTypeStr=single
  Data Type Conversion2 : DataTypeConversion  OutDataTypeStr=single
  Limis eval : MATLAB Function  TreatAsAtomicUnit=on
  Saturation Dynamic : simulink/Discontinuities/Saturation Dynamic  OutMin=[]  OutMax=[]  OutDataTypeStr=single  OutputDataTypeScalingMode=single  OutDataType=fixdt(1, 16)  OutScaling=2^-10  DoSatur=off
  ang Ace des : Outport
  wires:
  Limis eval/1(Limit_up) -> Data Type Conversion1/1
  Limis eval/2(Limit_down) -> Data Type Conversion2/1
  Ang Ace des/1 -> Saturation Dynamic/2, Limis eval/1(Ang_Accel)
  Data Type Conversion1/1 -> Saturation Dynamic/1
  Data Type Conversion2/1 -> Saturation Dynamic/3
  Saturation Dynamic/1 -> ang Ace des/1

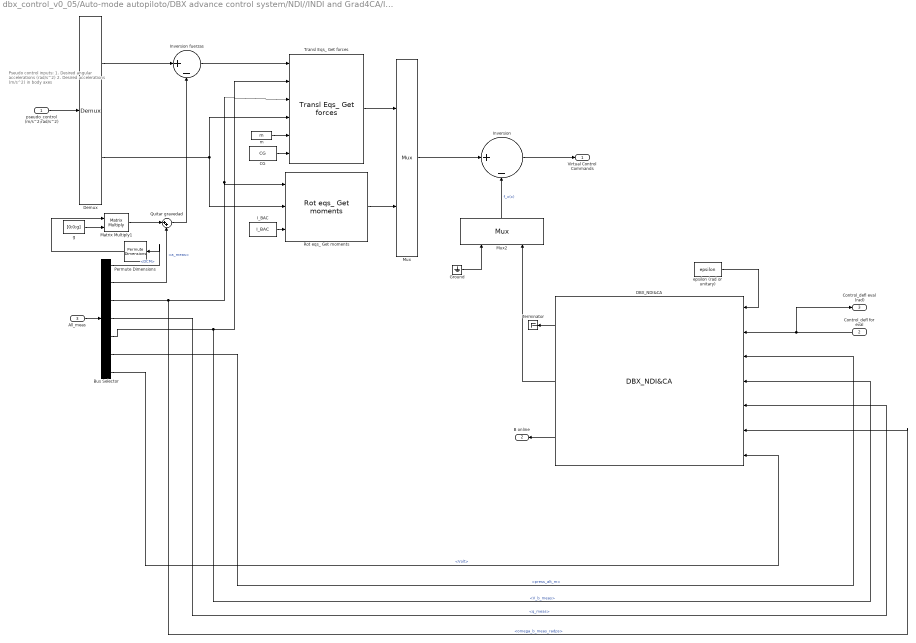
== system dbx_control_v0_05/Auto-mode autopiloto/DBX advance control system/NDI//INDI and Grad4CA/INDI and NDI ==
  note: Pseudo control inputs:
      | 1. Desired angular accelerations (rad/s^2)
      | 2. Desired accelerations (m/s^2) in body axes
  pseudo_control (m/s^2;rad/s^2) : Inport
  Control_defl for eval : Inport  Port=2
  All_meas : Inport  Port=3
  Bus Selector : BusSelector  OutputSignals=Params.DCM,Meas.a_meas,Meas.omega_b_meas_radps,Meas.q_meas,Meas.V_b_meas,Meas.press_alt_m,Meas.Volt
  CG : Constant  Value=CG
  DBX_NDI&CA : DBX_Control/DBX_NDI&CA  SystemSampleTime=-1
  Demux : Demux  Outputs=[3,3]
  Ground : Ground
  I_BAC : Constant  Value=I_BAC
  Inversion : Sum  Inputs=|+-
  Inversion fuerzas : Sum  Inputs=|+-
  Matrix Multiply1 : Product  Multiplication=Matrix(*)
  Mux : Mux  Inputs=[3,3]
  Mux2 : Mux  Inputs=[3,3]
  Permute Dimensions : PermuteDimensions
  Quitar gravedad : Sum  Inputs=|++
  Rot eqs_ Get moments : DBX_Control/Rot eqs_ Get moments
  Terminator : Terminator
  Transl Eqs_ Get forces : DBX_Control/Transl Eqs_ Get forces
  epsilon (rad or unitary) : Constant  Value=epsilon
  g : Constant  Value=[0;0;g]
  m : Constant  Value=m
  Virtual Control Commands : Outport
  B online : Outport  Port=2
  Control_defl eval (rad) : Outport  Port=3
  wires:
  DBX_NDI&CA/3 -> B online/1
  Mux/1 -> Inversion/1
  Mux2/1 -> Inversion/2  "f_x(x)"
  All_meas/1 -> Bus Selector/1
  pseudo_control (m/s^2;rad/s^2)/1 -> Demux/1
  Demux/2 -> Rot eqs_ Get moments/2, Transl Eqs_ Get forces/4
  Demux/1 -> Inversion fuerzas/1
  Bus Selector/3 -> Transl Eqs_ Get forces/3, Rot eqs_ Get moments/1, DBX_NDI&CA/6  "<omega_b_meas_radps>"
  Bus Selector/5 -> DBX_NDI&CA/4, Transl Eqs_ Get forces/2  "<V_b_meas>"
  Control_defl for eval/1 -> DBX_NDI&CA/2, Control_defl eval (rad)/1
  Bus Selector/6 -> DBX_NDI&CA/3  "<press_alt_m>"
  Bus Selector/4 -> DBX_NDI&CA/5  "<q_meas>"
  m/1 -> Transl Eqs_ Get forces/5
  epsilon (rad or unitary)/1 -> DBX_NDI&CA/1
  Transl Eqs_ Get forces/1 -> Mux/1
  Rot eqs_ Get moments/1 -> Mux/2
  DBX_NDI&CA/2 -> Mux2/2
  Inversion/1 -> Virtual Control Commands/1
  Bus Selector/7 -> DBX_NDI&CA/7  "<Volt>"
  I_BAC/1 -> Rot eqs_ Get moments/3
  CG/1 -> Transl Eqs_ Get forces/6
  Ground/1 -> Mux2/1
  Inversion fuerzas/1 -> Transl Eqs_ Get forces/1
  DBX_NDI&CA/1 -> Terminator/1
  Permute Dimensions/1 -> Matrix Multiply1/1
  g/1 -> Matrix Multiply1/2
  Bus Selector/2 -> Quitar gravedad/2  "<a_meas>"
  Quitar gravedad/1 -> Inversion fuerzas/2
  Matrix Multiply1/1 -> Quitar gravedad/1
  Bus Selector/1 -> Permute Dimensions/1  "<DCM>"

== system dbx_control_v0_05/Auto-mode autopiloto/DBX advance control system/NDI//INDI and Grad4CA/NDI ==
  note: Pseudo control inputs:
      | 1. Desired angular accelerations (rad/s^2)
      | 2. Desired accelerations (m/s^2) in body axes
  pseudo_control (m/s^2;rad/s^2) : Inport
  Control_defl for eval : Inport  Port=2
  All_meas : Inport  Port=3
  Bus Selector : BusSelector  OutputSignals=Meas.omega_b_meas_radps,Meas.q_meas,Meas.V_b_meas,Meas.press_alt_m,Meas.Volt
  CG : Constant  Value=CG
  DBX_NDI&CA : DBX_Control_lib/DBX_NDI&CA  SystemSampleTime=-1
  Demux : Demux  Outputs=[3,3]
  I_BAC : Constant  Value=I_BAC
  Inversion : Sum  Inputs=|+-
  Mux : Mux  Inputs=[3,3]
  Mux2 : Mux  Inputs=[3,3]
  Rot eqs_ Get moments : DBX_Control_lib/Rot eqs_ Get moments
  Transl Eqs_ Get forces : DBX_Control_lib/Transl Eqs_ Get forces
  epsilon (rad or unitary) : Constant  Value=epsilon
  m : Constant  Value=m
  Virtual Control Commands : Outport
  B online : Outport  Port=2
  Control_defl eval (rad) : Outport  Port=3
  wires:
  CG/1 -> Transl Eqs_ Get forces/6
  I_BAC/1 -> Rot eqs_ Get moments/3
  Bus Selector/5 -> DBX_NDI&CA/7  "<Volt>"
  Inversion/1 -> Virtual Control Commands/1
  DBX_NDI&CA/2 -> Mux2/2
  DBX_NDI&CA/1 -> Mux2/1
  Rot eqs_ Get moments/1 -> Mux/2
  Transl Eqs_ Get forces/1 -> Mux/1
  epsilon (rad or unitary)/1 -> DBX_NDI&CA/1
  m/1 -> Transl Eqs_ Get forces/5
  Bus Selector/2 -> DBX_NDI&CA/5  "<q_meas>"
  Bus Selector/4 -> DBX_NDI&CA/3  "<press_alt_m>"
  Control_defl for eval/1 -> Control_defl eval (rad)/1, DBX_NDI&CA/2
  Bus Selector/3 -> Transl Eqs_ Get forces/2, DBX_NDI&CA/4  "<V_b_meas>"
  Bus Selector/1 -> Rot eqs_ Get moments/1, Transl Eqs_ Get forces/3, DBX_NDI&CA/6  "<omega_b_meas_radps>"
  Demux/1 -> Transl Eqs_ Get forces/1
  Demux/2 -> Transl Eqs_ Get forces/4, Rot eqs_ Get moments/2
  pseudo_control (m/s^2;rad/s^2)/1 -> Demux/1
  All_meas/1 -> Bus Selector/1
  Mux2/1 -> Inversion/2  "f_x(x)"
  Mux/1 -> Inversion/1
  DBX_NDI&CA/3 -> B online/1

== system dbx_control_v0_05/Auto-mode autopiloto/DBX advance control system/NDI//INDI and Grad4CA/NDI incremental gradient ==
  note: Pseudo control inputs:
      | 1. Desired angular accelerations (rad/s^2)
      | 2. Desired accelerations (m/s^2) in body axes
  pseudo_control (m/s^2;rad/s^2) : Inport
  Control_defl for eval : Inport  Port=2
  All_meas : Inport  Port=3
  Bus Selector : BusSelector  OutputSignals=Meas.omega_b_meas_radps,Meas.q_meas,Meas.V_b_meas,Meas.press_alt_m,Meas.Volt
  CG : Constant  Value=CG  OutDataTypeStr=single
  DBX_NDI&CA Incremental Gradient : DBX_Control_lib/DBX_NDI&CA Incremental Gradient  SystemSampleTime=-1
  Demux : Demux  Outputs=[3,3]
  I_BAC : Constant  Value=I_BAC  OutDataTypeStr=single
  Inversion : Sum  Inputs=|+-
  Mux : Mux  Inputs=[3,3]
  Mux2 : Mux  Inputs=[3,3]
  Rot eqs_ Get moments : DBX_Control_lib/Rot eqs_ Get moments
  Transl Eqs_ Get forces : DBX_Control_lib/Transl Eqs_ Get forces
  epsilon (rad or unitary) : Constant  Value=epsilon  OutDataTypeStr=single
  m : Constant  Value=m  OutDataTypeStr=single
  Virtual Control Commands : Outport
  B online : Outport  Port=2
  Control_defl eval (rad) : Outport  Port=3
  wires:
  DBX_NDI&CA Incremental Gradient/3 -> B online/1
  Mux/1 -> Inversion/1
  Mux2/1 -> Inversion/2  "f_x(x)"
  All_meas/1 -> Bus Selector/1
  pseudo_control (m/s^2;rad/s^2)/1 -> Demux/1
  Demux/2 -> Rot eqs_ Get moments/2, Transl Eqs_ Get forces/4
  Demux/1 -> Transl Eqs_ Get forces/1
  Bus Selector/1 -> DBX_NDI&CA Incremental Gradient/6, Transl Eqs_ Get forces/3, Rot eqs_ Get moments/1  "<omega_b_meas_radps>"
  Bus Selector/3 -> DBX_NDI&CA Incremental Gradient/4, Transl Eqs_ Get forces/2  "<V_b_meas>"
  Control_defl for eval/1 -> DBX_NDI&CA Incremental Gradient/2, Control_defl eval (rad)/1
  Bus Selector/4 -> DBX_NDI&CA Incremental Gradient/3  "<press_alt_m>"
  Bus Selector/2 -> DBX_NDI&CA Incremental Gradient/5  "<q_meas>"
  m/1 -> Transl Eqs_ Get forces/5
  epsilon (rad or unitary)/1 -> DBX_NDI&CA Incremental Gradient/1
  Transl Eqs_ Get forces/1 -> Mux/1
  Rot eqs_ Get moments/1 -> Mux/2
  DBX_NDI&CA Incremental Gradient/1 -> Mux2/1
  DBX_NDI&CA Incremental Gradient/2 -> Mux2/2
  Inversion/1 -> Virtual Control Commands/1
  Bus Selector/5 -> DBX_NDI&CA Incremental Gradient/7  "<Volt>"
  I_BAC/1 -> Rot eqs_ Get moments/3
  CG/1 -> Transl Eqs_ Get forces/6

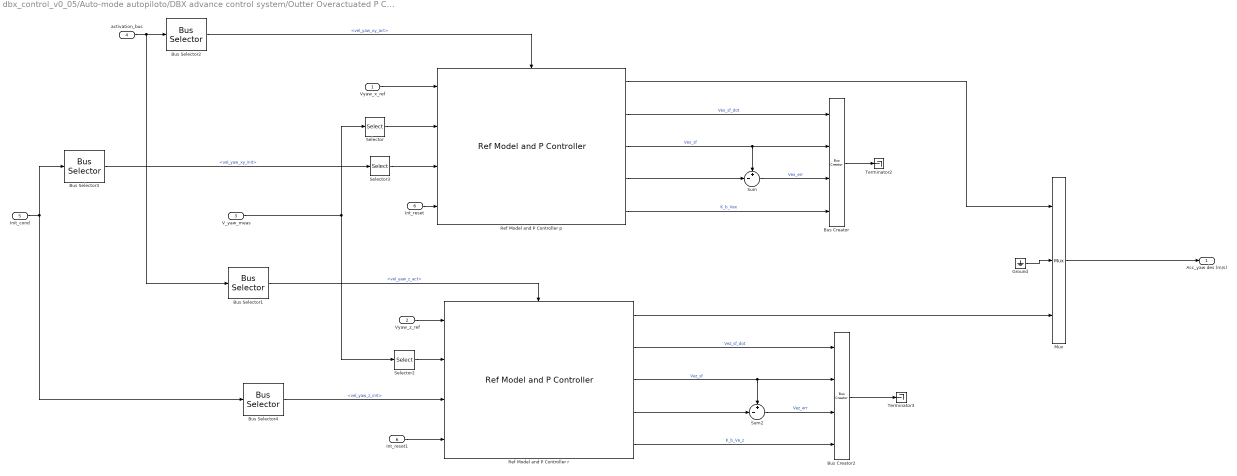
== system dbx_control_v0_05/Auto-mode autopiloto/DBX advance control system/Outter Overactuated P Controller/Velocity Controller ==
  Vyaw_x_ref : Inport
  Vyaw_z_ref : Inport  Port=2
  V_yaw_meas : Inport  Port=3
  activation_bus : Inport  Port=4
  Init_cond : Inport  Port=5
  Int_reset : Inport  Port=6
  Bus Creator : BusCreator
  Bus Creator2 : BusCreator
  Bus Selector1 : BusSelector  OutputSignals=vel_yaw_z_act
  Bus Selector2 : BusSelector  OutputSignals=vel_yaw_xy_act
  Bus Selector3 : BusSelector  OutputSignals=vel_yaw_xy_init
  Bus Selector4 : BusSelector  OutputSignals=vel_yaw_z_init
  Ground : Ground
  Int_reset1 : InportShadow  Port=6
  Mux : Mux  Inputs=3
  Ref Model and P Controller p : DBX_Control_lib/Ref Model and P Controller  tau=2  RisingSlewLimit=1  FallingSlewLimit=-1  K_f=0.5  K_b=1
  Ref Model and P Controller r : DBX_Control_lib/Ref Model and P Controller  tau=1  RisingSlewLimit=1  FallingSlewLimit=-1  K_f=0.4  K_b=8
  Selector : Selector  InputPortWidth=3
  Selector2 : Selector  InputPortWidth=3  Indices=3
  Selector3 : Selector  InputPortWidth=2
  Sum : Sum  Inputs=+-|
  Sum2 : Sum  Inputs=+-|
  Terminator2 : Terminator
  Terminator3 : Terminator
  Acc_yaw des (m/s) : Outport
  wires:
  Ref Model and P Controller r/5 -> Bus Creator2/4  "K_b_Ve_z"
  Ref Model and P Controller r/4 -> Sum2/2
  Sum2/1 -> Bus Creator2/3  "Vez_err"
  Ref Model and P Controller r/3 -> Bus Creator2/2, Sum2/1  "Vez_sf"
  Ref Model and P Controller r/2 -> Bus Creator2/1  "Vez_sf_dot"
  Ref Model and P Controller p/5 -> Bus Creator/4  "K_b_Vex"
  Ref Model and P Controller p/4 -> Sum/2
  Selector2/1 -> Ref Model and P Controller r/2
  Bus Creator2/1 -> Terminator3/1
  Bus Creator/1 -> Terminator2/1
  Sum/1 -> Bus Creator/3  "Vex_err"
  Ref Model and P Controller p/3 -> Bus Creator/2, Sum/1  "Vex_sf"
  Ref Model and P Controller p/2 -> Bus Creator/1  "Vex_sf_dot"
  Ref Model and P Controller r/1 -> Mux/3
  Vyaw_z_ref/1 -> Ref Model and P Controller r/1
  Mux/1 -> Acc_yaw des (m/s)/1
  Ref Model and P Controller p/1 -> Mux/1
  Vyaw_x_ref/1 -> Ref Model and P Controller p/1
  V_yaw_meas/1 -> Selector/1, Selector2/1
  Selector/1 -> Ref Model and P Controller p/2
  activation_bus/1 -> Bus Selector1/1, Bus Selector2/1
  Bus Selector2/1 -> Ref Model and P Controller p/Enable  "<vel_yaw_xy_act>"
  Bus Selector1/1 -> Ref Model and P Controller r/Enable  "<vel_yaw_z_act>"
  Init_cond/1 -> Bus Selector4/1, Bus Selector3/1
  Bus Selector3/1 -> Selector3/1  "<vel_yaw_xy_init>"
  Selector3/1 -> Ref Model and P Controller p/3
  Bus Selector4/1 -> Ref Model and P Controller r/3  "<vel_yaw_z_init>"
  Ground/1 -> Mux/2
  Int_reset1/1 -> Ref Model and P Controller r/4
  Int_reset/1 -> Ref Model and P Controller p/4

== matlab function dbx_control_v0_05/Manual flight mode/MATLAB Function1 ==
  data: Euler_dot input size=[3,1]; Omega output; euler_ang input size=[3,1]
function Omega = Euler_dot_2_omega(Euler_dot,euler_ang)

phi = euler_ang(1);
theta = euler_ang(2);


A = [1          0               -sin(theta)         ;
     0          cos(phi)        sin(phi)*cos(theta) ;
     0          -sin(phi)       cos(phi)*cos(theta)];

Omega = A*Euler_dot ;

== matlab function dbx_control_v0_05/Px4_to_simulink input interface/Px4_to_simulink input interface/MATLAB Function ==
  data: T_yaw output; yaw input
function T_yaw = Yaw_rotate(yaw)


T_yaw=[cos(yaw),    sin(yaw),   0;
        -sin(yaw),  cos(yaw),   0;
        0,      0,              1];

== matlab function dbx_control_v0_05/Manual flight mode/pwm_out1 ==
  data: Roll input; M1 output size=1; P input size=1; Y input size=1; T input size=1; M2 output size=1; M3 output size=1; S3 output size=1; R parameter
function [M1, M2, M3, S3] = motor_mixer(Roll, P, Y, T,R)
%% Salidas de Throtle de -1 a 1 y angulos en rad
% idle_motor = 0;

% DBX

M1 = single(max(T+Roll/2+P/3,0));
M2 = single(max(T-Roll/2+P/3,0));
M3 = single(max(T-2*P/3,0));


S3 = single(0.3*R/(max(T-2*P/3,0.2))*(T-Y)) ;

% Quad X
% M1 = ((Roll + Pitch - Yaw) / 2 * Thrust + Thrust) * 1000 + idle_motor;
% M2 = ((-Roll + Pitch + Yaw) / 2 * Thrust + Thrust) * 1000 + idle_motor;
% M3 = ((-Roll - Pitch - Yaw) / 2 * Thrust + Thrust) * 1000 + idle_motor;
% S3 = ((Roll - Pitch + Yaw) / 2 * Thrust + Thrust) * 1000 + idle_motor;
% M5 = 1000;
% M6 = 1000;
% M7 = 1000;
% M8 = 1000;

% Quad +
% M1 = ((Pitch - Yaw) * Thrust / 2 + Thrust) * 1000 + idle_PWM;
% M2 = ((-Roll + Yaw) * Thrust / 2 + Thrust) * 1000 + idle_PWM;
% M3 = ((-Pitch - Yaw) * Thrust / 2 + Thrust) * 1000 + idle_PWM;
% M4 = ((Roll + Yaw) * Thrust / 2 + Thrust) * 1000 + idle_PWM;
% M5 = 1000;
% M6 = 1000;
% M7 = 1000;
% M8 = 1000;

% Hex X
% M1 = ((Pitch + Roll / 2 - Yaw) * Thrust / 2 + Thrust) * 1000 + idle_PWM;
% M2 = ((Pitch - Roll / 2 + Yaw) * Thrust / 2 + Thrust) * 1000 + idle_PWM;
% M3 = ((-Roll - Yaw) * Thrust / 2 + Thrust) * 1000 + idle_PWM;
% M4 = ((-Pitch - Roll / 2 + Yaw) * Thrust / 2 + Thrust) * 1000 + idle_PWM;
% M5 = ((-Pitch + Roll / 2 - Yaw) * Thrust / 2 + Thrust) * 1000 + idle_PWM;
% M6 = ((Roll + Yaw) * Thrust / 2 + Thrust) * 1000 + idle_PWM;
% M7 = 1000;
% M8 = 1000;


end

== matlab function dbx_control_v0_05/Auto-mode autopiloto/DBX advance control system/Inner PI Controller Euler/MATLAB Function ==
  data: omega_b input size=[3,1]; Euler_dot output; Euler input size=[3,1]
function Euler_dot = omega2Euler_dot(omega_b,Euler)

phi = Euler(1);
theta = Euler(2);
psi = Euler(3);


A = [1          0               -sin(theta)         ;
     0          cos(phi)        sin(phi)*cos(theta) ;
     0          -sin(phi)       cos(phi)*cos(theta)];

Euler_dot = A'*omega_b ;

== matlab function dbx_control_v0_05/Auto-mode autopiloto/DBX advance control system/Inner PI Controller Euler/MATLAB Function1 ==
  data: Euler_dot input size=[3,1]; Omega output; euler_ang input size=[3,1]
function Omega = Euler_dot_2_omega(Euler_dot,euler_ang)

phi = euler_ang(1);
theta = euler_ang(2);
psi = euler_ang(3);


A = [1          0               -sin(theta)         ;
     0          cos(phi)        sin(phi)*cos(theta) ;
     0          -sin(phi)       cos(phi)*cos(theta)];

Omega = A*Euler_dot ;

== matlab function dbx_control_v0_05/Auto-mode autopiloto/DBX advance control system/Inner PI Controller Euler/Limits in Ang accel/Limis eval ==
  data: Ang_Accel input size=[3,1]; Limit_up output; Limit_down output; A_M parameter; L_M parameter; m parameter; g parameter; I_BAC parameter
function [Limit_up,Limit_down]= Max_ang_accels(Ang_Accel,A_M,L_M,m,g,I_BAC)

Limit_up=Ang_Accel;
Limit_down=Ang_Accel;

Limit_up(1) =   abs( (2*m*g/3*A_M/2  )/I_BAC(1,1)  )* 1 ;
Limit_down(1) = -Limit_up(1) ;

Limit_up(2) = abs(1/3*L_M*m*g*2/3)/I_BAC(2,2)* 1 ;
Limit_down(2) = -Limit_up(2);


Limit_up(3) = ( 2/3*L_M*m*g/3*sin(15/180*pi) )/I_BAC(3,3)* 1 ;
Limit_down(3) = -Limit_up(3) ;
